simulink model "Supported_and_unsupported_combinations"  (Simulink 7.8)
settings: Solver=ode15s  StartTime=0.0  StopTime=inf  MaxStep=0.2  RelTol=1e-3
undefined symbols (not defined in the file): Engine, Engine1, Engine2, Engine3, Engine4, Engine5, Engine6, Engine7, Engine8, Engine9
libraries: sFunctionBlocks x32
(part 4 of 4)

== system Supported_and_unsupported_combinations/Engine8/IntakeManifold ==
  Mout : Inport
  inflow : Inport  Port=2
  IsothermalManifoldXO2 : S-Function  FunctionName=orsb_reservoir_isothermal_XO2  Parameters=V , R , Cp , pinit , XO2init ,  EnableBusSupport=off  mask(reservoir isothermal XO2 ){V=41.2801, R=288.4, Cp=1020, pinit=205590, XO2init=0.22}
      mask prompts: V "reservoir volume [l]"; R "gas constant [J/K/kg]"; Cp "fixed pressure spec heat [J/kg/K]"; pinit "initial pressure [Pa]"; XO2init "initial oxygen mass fraction [-]"
      mask help: Isothermal reservoir model with pressure and oxygen mass fraction as internal states.
      mask TabNameString: General ,General ,General ,Initialization ,Initialization
      mask Display:
      | port_label('input', 1, 'min ');
      | port_label('input', 2, 'mout ');
      | port_label('input', 3, 'Tin ');
      | port_label('input', 4, 'O2min ');
      | port_label('output', 1, 'pout ');
      | port_label('output', 2, 'XO2out ');
  Pim : Outport
  XO2out : Outport  Port=2
  outflow : Outport  Port=3
  tag scope: EngineIntakeManifold_OutletPressure=global
  wires:
  Mout/1 -> IsothermalManifoldXO2/2
  IsothermalManifoldXO2/1 -> Pim/1, [EngineIntakeManifold_OutletPressure]
  IsothermalManifoldXO2/2 -> XO2out/1
  inflow/1 -> outflow/1  "flow"
  [MixTotalInFlow_Massflow] -> IsothermalManifoldXO2/1
  [MixTotalInFlow_OxygenFlow] -> IsothermalManifoldXO2/4
  [MixTotalInFlow_MixtureTemperature] -> IsothermalManifoldXO2/3

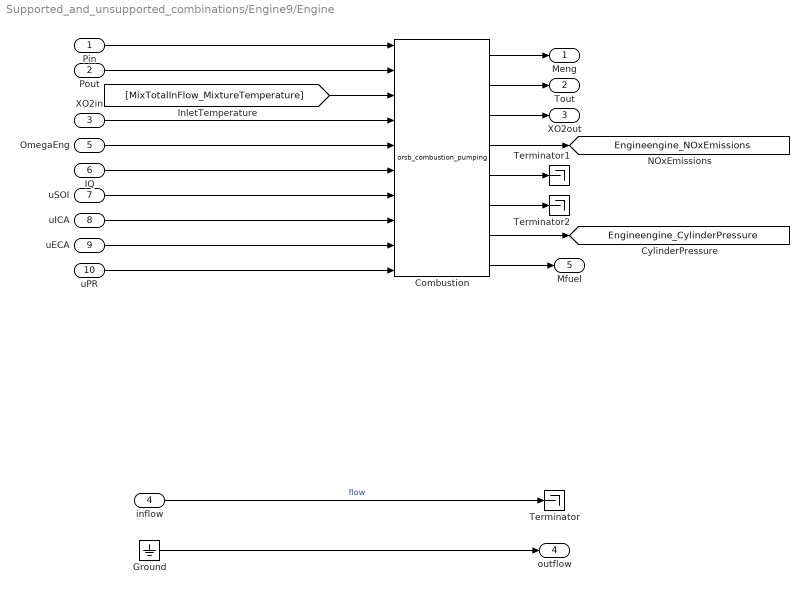
== system Supported_and_unsupported_combinations/Engine9/Engine ==
  Pin : Inport
  Pout : Inport  Port=2
  XO2in : Inport  Port=3
  inflow : Inport  Port=4
  OmegaEng : Inport  Port=5
  IQ : Inport  Port=6
  uSOI : Inport  Port=7
  uICA : Inport  Port=8
  uECA : Inport  Port=9
  uPR : Inport  Port=10
  Combustion : S-Function  FunctionName=orsb_combustion_pumping  Parameters=Displ, CompRatio, Ncyl, ValveMdl, TmpMdl, IgnitMdl, PressMdl, Cp, Cv, port_num_NOx, NOxMdl,  EnableBusSupport=off  mask(combustion_pumping){Displ=12.9, CompRatio=18, Ncyl=6, ValveMdl=[0.00961171539106083 -0.172384589641163], TmpMdl=[-0.025503095647334 0.175522235872159 0.0255043476751577 0.0373865335774022 0], IgnitMdl=[0.484351292851209 0.143524113288744 -0.055676015193126 -0.0109937044135945 -0.025686692856836], PressMdl=[5.48733176777509 -0.092135251339445 -0.0332005633970498 0.773921335537747], Cp=1500, Cv=1200, port_num_NOx=4, NOxMdl=[-0.0710772115732251 13.258266248882 2.53650929146028 -4.98871540780321 18.9690745540948 3.51983329140351 7.35640722696346 -29.5494146545499 -12.7663876549855 -0.0214097840965915 0.143608010417368 -1.21453634962735 0.541720620436424 -0.0774873942784366 -0.515304310267613]}
      mask prompts: Displ "displacement"; CompRatio "compression ratio"; Ncyl "number of cylinders"; ValveMdl "valve model"; TmpMdl "temperature model"; IgnitMdl "ignition model"; PressMdl "pressure model"; port_num_NOx "Model NOx output port number"; NOxMdl "NOx parameters"
      mask help: Combustion development
      mask TabNameString: geometry,geometry,geometry,thermodynamics,thermodynamics,thermodynamics,thermodynamics,thermodynamics,thermodynamics,NOx,NOx
      mask Display:
      | port_label('input', 1, 'Pi');
      | port_label('input', 2, 'Pe');
      | port_label('input', 3, 'Ti');
      | port_label('input', 4, 'O2i');
      | port_label('input', 5, 'Ne');
      | port_label('input', 6, 'iq');
      | port_label('input', 7, 'soi');
      | port_label('input', 8, 'ica');
      | port_label('input', 9, 'eca');
      | port_label('input', 10, 'Prail');
      | port_label('output', 1, 'M');
      | port_label('output', 2, 'Te');
      | port_label('output', 3, 'XO2e');
      | port_label('output', 4, 'NOx');
      | port_label('output', 5, 'lambda');
      | port_label('output', 6, 'phi_ign');
      | port_label('output', 7, 'Pcyl');
      | port_label('output', 8, 'Mf');
  Ground : Ground
  Terminator : Terminator
  Terminator1 : Terminator
  Terminator2 : Terminator
  Meng : Outport
  Tout : Outport  Port=2
  XO2out : Outport  Port=3
  outflow : Outport  Port=4
  Mfuel : Outport  Port=5
  tag scope: Engineengine_CylinderPressure=global, Engineengine_NOxEmissions=global
  wires:
  uSOI/1 -> Combustion/7
  [MixTotalInFlow_MixtureTemperature] -> Combustion/3
  Combustion/4 -> [Engineengine_NOxEmissions]
  XO2in/1 -> Combustion/4
  Combustion/3 -> XO2out/1
  Combustion/2 -> Tout/1
  Pout/1 -> Combustion/2
  Pin/1 -> Combustion/1
  OmegaEng/1 -> Combustion/5
  Ground/1 -> outflow/1
  inflow/1 -> Terminator/1  "flow"
  Combustion/1 -> Meng/1
  Combustion/5 -> Terminator1/1
  Combustion/6 -> Terminator2/1
  Combustion/7 -> [Engineengine_CylinderPressure]
  Combustion/8 -> Mfuel/1
  IQ/1 -> Combustion/6
  uICA/1 -> Combustion/8
  uECA/1 -> Combustion/9
  uPR/1 -> Combustion/10

== system Supported_and_unsupported_combinations/Engine9/ExhaustManifold ==
  Meng : Inport
  Tin : Inport  Port=2
  XO2in : Inport  Port=3
  inflow : Inport  Port=4
  Mfuel : Inport  Port=5
  Add4 : Sum
  AdiabaticManifoldXO2 : S-Function  FunctionName=orsb_reservoir_adiabatic_XO2  Parameters=V , R , Cp , pinit , Tinit , XO2init ,  EnableBusSupport=off  mask(reservoir adiabatic XO2 ){V=50, R=288.4, Cp=1135, pinit=247140, Tinit=720.22, XO2init=0.15}
      mask prompts: V "reservoir volume [l]"; R "gas constant [J/K/kg]"; Cp "fixed pressure spec heat [J/kg/K]"; pinit "initial pressure [Pa]"; Tinit "initial temperature [K]"; XO2init "initial oxygen mass fraction [-]"
      mask help: Adiabatic reservoir model with pressure, temperature, and oxygen mass fraction as internal states.
      mask TabNameString: General ,General ,General ,Initialization ,Initialization ,Initialization
      mask Display:
      | port_label('input', 1, 'min ');
      | port_label('input', 2, 'mout ');
      | port_label('input', 3, 'Tin ');
      | port_label('input', 4, 'O2min ');
      | port_label('output', 1, 'pout ');
      | port_label('output', 2, 'Tout ');
      | port_label('output', 3, 'XO2out ');
  Conversion_XO2_lambda : Fcn  Expr=u(1) / 0.231362 * (1 + 14.59) / (14.59 * (1 - u(1) / 0.231362))+1
  Product2 : Product  RndMeth=Zero
  Saturation : Saturate  UpperLimit=0.2313  LowerLimit=0
  Pout : Outport
  outflow : Outport  Port=2
  tag scope: EngineExhaustManifold_OutletLambda=global, EngineExhaustManifold_OutletOxygenFraction=global, EngineExhaustManifold_OutletPressure=global, EngineExhaustManifold_OutletTemperature=global
  wires:
  Conversion_XO2_lambda/1 -> [EngineExhaustManifold_OutletLambda]
  [FlowSplitterTotalOutFlow_Massflow] -> AdiabaticManifoldXO2/2
  Mfuel/1 -> Add4/1
  inflow/1 -> outflow/1  "flow"
  XO2in/1 -> Product2/2
  AdiabaticManifoldXO2/3 -> [EngineExhaustManifold_OutletOxygenFraction], Saturation/1
  Tin/1 -> AdiabaticManifoldXO2/3
  AdiabaticManifoldXO2/2 -> [EngineExhaustManifold_OutletTemperature]
  AdiabaticManifoldXO2/1 -> [EngineExhaustManifold_OutletPressure], Pout/1
  Meng/1 -> Add4/2
  Product2/1 -> AdiabaticManifoldXO2/4
  Add4/1 -> Product2/1, AdiabaticManifoldXO2/1
  Saturation/1 -> Conversion_XO2_lambda/1

== system Supported_and_unsupported_combinations/Engine9/IntakeManifold ==
  Mout : Inport
  inflow : Inport  Port=2
  IsothermalManifoldXO2 : S-Function  FunctionName=orsb_reservoir_isothermal_XO2  Parameters=V , R , Cp , pinit , XO2init ,  EnableBusSupport=off  mask(reservoir isothermal XO2 ){V=41.2801, R=288.4, Cp=1020, pinit=205590, XO2init=0.22}
      mask prompts: V "reservoir volume [l]"; R "gas constant [J/K/kg]"; Cp "fixed pressure spec heat [J/kg/K]"; pinit "initial pressure [Pa]"; XO2init "initial oxygen mass fraction [-]"
      mask help: Isothermal reservoir model with pressure and oxygen mass fraction as internal states.
      mask TabNameString: General ,General ,General ,Initialization ,Initialization
      mask Display:
      | port_label('input', 1, 'min ');
      | port_label('input', 2, 'mout ');
      | port_label('input', 3, 'Tin ');
      | port_label('input', 4, 'O2min ');
      | port_label('output', 1, 'pout ');
      | port_label('output', 2, 'XO2out ');
  Pim : Outport
  XO2out : Outport  Port=2
  outflow : Outport  Port=3
  tag scope: EngineIntakeManifold_OutletPressure=global
  wires:
  [MixTotalInFlow_MixtureTemperature] -> IsothermalManifoldXO2/3
  [MixTotalInFlow_OxygenFlow] -> IsothermalManifoldXO2/4
  [MixTotalInFlow_Massflow] -> IsothermalManifoldXO2/1
  inflow/1 -> outflow/1  "flow"
  IsothermalManifoldXO2/2 -> XO2out/1
  IsothermalManifoldXO2/1 -> [EngineIntakeManifold_OutletPressure], Pim/1
  Mout/1 -> IsothermalManifoldXO2/2

== system Supported_and_unsupported_combinations/FlowSplitter/OutFlow1 ==
  inflow : Inport
  Mout1 : Outport
  outflow : Outport  Port=2
  tag scope: none=global
  wires:
  inflow/1 -> outflow/1  "flow"
  [none] -> [none], Mout1/1

== system Supported_and_unsupported_combinations/FlowSplitter/OutFlow2 ==
  inflow : Inport
  Mout2 : Outport
  outflow : Outport  Port=2
  tag scope: none=global
  wires:
  [none] -> [none], Mout2/1
  inflow/1 -> outflow/1  "flow"

== system Supported_and_unsupported_combinations/FlowSplitter/TotalOutFlow ==
  Mout1 : Inport
  Mout2 : Inport  Port=2
  inflow : Inport  Port=3
  AuxiliaryManifold : sFunctionBlocks/AuxiliaryManifold  Tag=isAuxManifold  V=1  R=288  Cp=1020  pinit=1e5  isActive=0
  FlowSummation : Sum
  outflow : Outport
  tag scope: none=global
  wires:
  [none] -> AuxiliaryManifold/3
  [none] -> AuxiliaryManifold/1
  AuxiliaryManifold/1 -> [none]
  inflow/1 -> outflow/1  "flow"
  Mout1/1 -> FlowSummation/1
  Mout2/1 -> FlowSummation/2
  FlowSummation/1 -> AuxiliaryManifold/2, [none]

== system Supported_and_unsupported_combinations/FlowSplitter1/OutFlow1 ==
  inflow : Inport
  Mout1 : Outport
  outflow : Outport  Port=2
  tag scope: none=global
  wires:
  [none] -> Mout1/1, [none]
  inflow/1 -> outflow/1  "flow"

== system Supported_and_unsupported_combinations/FlowSplitter1/OutFlow2 ==
  inflow : Inport
  Mout2 : Outport
  outflow : Outport  Port=2
  tag scope: none=global
  wires:
  inflow/1 -> outflow/1  "flow"
  [none] -> Mout2/1, [none]

== system Supported_and_unsupported_combinations/FlowSplitter1/TotalOutFlow ==
  Mout1 : Inport
  Mout2 : Inport  Port=2
  inflow : Inport  Port=3
  AuxiliaryManifold : sFunctionBlocks/AuxiliaryManifold  Tag=isAuxManifold  V=1  R=288  Cp=1020  pinit=1e5  isActive=0
  FlowSummation : Sum
  outflow : Outport
  tag scope: none=global
  wires:
  FlowSummation/1 -> [none], AuxiliaryManifold/2
  Mout2/1 -> FlowSummation/2
  Mout1/1 -> FlowSummation/1
  inflow/1 -> outflow/1  "flow"
  AuxiliaryManifold/1 -> [none]
  [none] -> AuxiliaryManifold/1
  [none] -> AuxiliaryManifold/3

== system Supported_and_unsupported_combinations/FlowSplitter2/OutFlow1 ==
  inflow : Inport
  Mout1 : Outport
  outflow : Outport  Port=2
  tag scope: none=global
  wires:
  [none] -> Mout1/1, [none]
  inflow/1 -> outflow/1  "flow"

== system Supported_and_unsupported_combinations/FlowSplitter2/OutFlow2 ==
  inflow : Inport
  Mout2 : Outport
  outflow : Outport  Port=2
  tag scope: none=global
  wires:
  inflow/1 -> outflow/1  "flow"
  [none] -> Mout2/1, [none]

== system Supported_and_unsupported_combinations/FlowSplitter2/TotalOutFlow ==
  Mout1 : Inport
  Mout2 : Inport  Port=2
  inflow : Inport  Port=3
  AuxiliaryManifold : sFunctionBlocks/AuxiliaryManifold  Tag=isAuxManifold  V=1  R=288  Cp=1020  pinit=1e5  isActive=0
  FlowSummation : Sum
  outflow : Outport
  tag scope: none=global
  wires:
  FlowSummation/1 -> [none], AuxiliaryManifold/2
  Mout2/1 -> FlowSummation/2
  Mout1/1 -> FlowSummation/1
  inflow/1 -> outflow/1  "flow"
  AuxiliaryManifold/1 -> [none]
  [none] -> AuxiliaryManifold/1
  [none] -> AuxiliaryManifold/3

== system Supported_and_unsupported_combinations/FlowSplitter3/OutFlow1 ==
  inflow : Inport
  Mout1 : Outport
  outflow : Outport  Port=2
  tag scope: none=global
  wires:
  inflow/1 -> outflow/1  "flow"
  [none] -> [none], Mout1/1

== system Supported_and_unsupported_combinations/FlowSplitter3/OutFlow2 ==
  inflow : Inport
  Mout2 : Outport
  outflow : Outport  Port=2
  tag scope: none=global
  wires:
  [none] -> [none], Mout2/1
  inflow/1 -> outflow/1  "flow"

== system Supported_and_unsupported_combinations/FlowSplitter3/TotalOutFlow ==
  Mout1 : Inport
  Mout2 : Inport  Port=2
  inflow : Inport  Port=3
  AuxiliaryManifold : sFunctionBlocks/AuxiliaryManifold  Tag=isAuxManifold  V=1  R=288  Cp=1020  pinit=1e5  isActive=0
  FlowSummation : Sum
  outflow : Outport
  tag scope: none=global
  wires:
  [none] -> AuxiliaryManifold/3
  [none] -> AuxiliaryManifold/1
  AuxiliaryManifold/1 -> [none]
  inflow/1 -> outflow/1  "flow"
  Mout1/1 -> FlowSummation/1
  Mout2/1 -> FlowSummation/2
  FlowSummation/1 -> AuxiliaryManifold/2, [none]

== system Supported_and_unsupported_combinations/Mix/InFlow1 ==
  inflow : Inport
  Flow1 : Subsystem
  Tin : Outport
  Min : Outport  Port=2
  XO2in : Outport  Port=3
  outflow : Outport  Port=4
  wires:
  Flow1/3(XO2in) -> XO2in/1
  Flow1/2(Min) -> Min/1
  Flow1/1(Tin) -> Tin/1
  inflow/1 -> outflow/1  "flow"
  [none] -> Flow1/3(In3)
  [none] -> Flow1/2(In2)
  [none] -> Flow1/1(In1)

== system Supported_and_unsupported_combinations/Mix/InFlow2 ==
  inflow : Inport
  Flow2 : Subsystem
  Tin : Outport
  Min : Outport  Port=2
  XO2in : Outport  Port=3
  outflow : Outport  Port=4
  wires:
  Flow2/3(XO2in) -> XO2in/1
  Flow2/2(Min) -> Min/1
  Flow2/1(Tin) -> Tin/1
  inflow/1 -> outflow/1  "flow"
  [none] -> Flow2/3(In3)
  [none] -> Flow2/2(In2)
  [none] -> Flow2/1(In1)

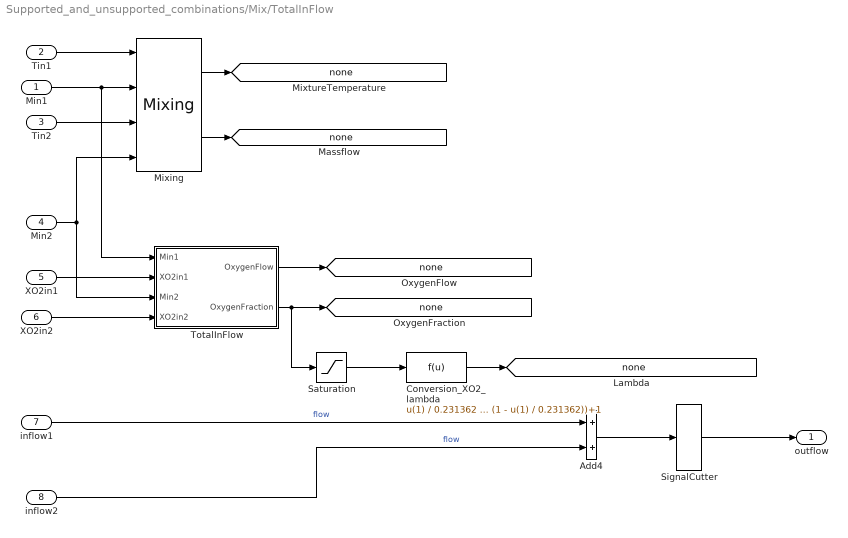
== system Supported_and_unsupported_combinations/Mix/TotalInFlow ==
  Min1 : Inport
  Tin1 : Inport  Port=2
  Tin2 : Inport  Port=3
  Min2 : Inport  Port=4
  XO2in1 : Inport  Port=5
  XO2in2 : Inport  Port=6
  inflow1 : Inport  Port=7
  inflow2 : Inport  Port=8
  Add4 : Sum
  Conversion_XO2_lambda : Fcn  Expr=u(1) / 0.231362 * (1 + 14.59) / (14.59 * (1 - u(1) / 0.231362))+1
  Mixing : sFunctionBlocks/Mixing  Cp1=1020.25  Cp2=1135.841
  Saturation : Saturate  UpperLimit=0.2313  LowerLimit=0
  SignalCutter : sFunctionBlocks/SignalCutter
  TotalInFlow : Subsystem
  outflow : Outport
  tag scope: none=global
  wires:
  SignalCutter/1 -> outflow/1
  Saturation/1 -> Conversion_XO2_lambda/1
  Conversion_XO2_lambda/1 -> [none]
  TotalInFlow/2(OxygenFraction) -> Saturation/1, [none]
  TotalInFlow/1(OxygenFlow) -> [none]
  inflow2/1 -> Add4/2  "flow"
  inflow1/1 -> Add4/1  "flow"
  Add4/1 -> SignalCutter/1
  XO2in2/1 -> TotalInFlow/4(XO2in2)
  XO2in1/1 -> TotalInFlow/2(XO2in1)
  Tin2/1 -> Mixing/3
  Tin1/1 -> Mixing/1
  Mixing/2 -> [none]
  Mixing/1 -> [none]
  Min2/1 -> TotalInFlow/3(Min2), Mixing/4
  Min1/1 -> TotalInFlow/1(Min1), Mixing/2

== system Supported_and_unsupported_combinations/Mix1/InFlow1 ==
  inflow : Inport
  Flow1 : Subsystem
  Tin : Outport
  Min : Outport  Port=2
  XO2in : Outport  Port=3
  outflow : Outport  Port=4
  wires:
  [none] -> Flow1/1(In1)
  [none] -> Flow1/2(In2)
  [none] -> Flow1/3(In3)
  inflow/1 -> outflow/1  "flow"
  Flow1/1(Tin) -> Tin/1
  Flow1/2(Min) -> Min/1
  Flow1/3(XO2in) -> XO2in/1

== system Supported_and_unsupported_combinations/Mix1/InFlow2 ==
  inflow : Inport
  Flow2 : Subsystem
  Tin : Outport
  Min : Outport  Port=2
  XO2in : Outport  Port=3
  outflow : Outport  Port=4
  wires:
  [none] -> Flow2/1(In1)
  [none] -> Flow2/2(In2)
  [none] -> Flow2/3(In3)
  inflow/1 -> outflow/1  "flow"
  Flow2/1(Tin) -> Tin/1
  Flow2/2(Min) -> Min/1
  Flow2/3(XO2in) -> XO2in/1

== system Supported_and_unsupported_combinations/Mix1/TotalInFlow ==
  Min1 : Inport
  Tin1 : Inport  Port=2
  Tin2 : Inport  Port=3
  Min2 : Inport  Port=4
  XO2in1 : Inport  Port=5
  XO2in2 : Inport  Port=6
  inflow1 : Inport  Port=7
  inflow2 : Inport  Port=8
  Add4 : Sum
  Conversion_XO2_lambda : Fcn  Expr=u(1) / 0.231362 * (1 + 14.59) / (14.59 * (1 - u(1) / 0.231362))+1
  Mixing : sFunctionBlocks/Mixing  Cp1=1020.25  Cp2=1135.841
  Saturation : Saturate  UpperLimit=0.2313  LowerLimit=0
  SignalCutter : sFunctionBlocks/SignalCutter
  TotalInFlow : Subsystem
  outflow : Outport
  tag scope: none=global
  wires:
  Min1/1 -> Mixing/2, TotalInFlow/1(Min1)
  Min2/1 -> Mixing/4, TotalInFlow/3(Min2)
  Mixing/1 -> [none]
  Mixing/2 -> [none]
  Tin1/1 -> Mixing/1
  Tin2/1 -> Mixing/3
  XO2in1/1 -> TotalInFlow/2(XO2in1)
  XO2in2/1 -> TotalInFlow/4(XO2in2)
  Add4/1 -> SignalCutter/1
  inflow1/1 -> Add4/1  "flow"
  inflow2/1 -> Add4/2  "flow"
  TotalInFlow/1(OxygenFlow) -> [none]
  TotalInFlow/2(OxygenFraction) -> [none], Saturation/1
  Conversion_XO2_lambda/1 -> [none]
  Saturation/1 -> Conversion_XO2_lambda/1
  SignalCutter/1 -> outflow/1

== system Supported_and_unsupported_combinations/Mix2/InFlow1 ==
  inflow : Inport
  Flow1 : Subsystem
  Tin : Outport
  Min : Outport  Port=2
  XO2in : Outport  Port=3
  outflow : Outport  Port=4
  wires:
  [none] -> Flow1/1(In1)
  [none] -> Flow1/2(In2)
  [none] -> Flow1/3(In3)
  inflow/1 -> outflow/1  "flow"
  Flow1/1(Tin) -> Tin/1
  Flow1/2(Min) -> Min/1
  Flow1/3(XO2in) -> XO2in/1

== system Supported_and_unsupported_combinations/Mix2/InFlow2 ==
  inflow : Inport
  Flow2 : Subsystem
  Tin : Outport
  Min : Outport  Port=2
  XO2in : Outport  Port=3
  outflow : Outport  Port=4
  wires:
  [none] -> Flow2/1(In1)
  [none] -> Flow2/2(In2)
  [none] -> Flow2/3(In3)
  inflow/1 -> outflow/1  "flow"
  Flow2/1(Tin) -> Tin/1
  Flow2/2(Min) -> Min/1
  Flow2/3(XO2in) -> XO2in/1

== system Supported_and_unsupported_combinations/Mix2/TotalInFlow ==
  Min1 : Inport
  Tin1 : Inport  Port=2
  Tin2 : Inport  Port=3
  Min2 : Inport  Port=4
  XO2in1 : Inport  Port=5
  XO2in2 : Inport  Port=6
  inflow1 : Inport  Port=7
  inflow2 : Inport  Port=8
  Add4 : Sum
  Conversion_XO2_lambda : Fcn  Expr=u(1) / 0.231362 * (1 + 14.59) / (14.59 * (1 - u(1) / 0.231362))+1
  Mixing : sFunctionBlocks/Mixing  Cp1=1020.25  Cp2=1135.841
  Saturation : Saturate  UpperLimit=0.2313  LowerLimit=0
  SignalCutter : sFunctionBlocks/SignalCutter
  TotalInFlow : Subsystem
  outflow : Outport
  tag scope: none=global
  wires:
  Min1/1 -> Mixing/2, TotalInFlow/1(Min1)
  Min2/1 -> Mixing/4, TotalInFlow/3(Min2)
  Mixing/1 -> [none]
  Mixing/2 -> [none]
  Tin1/1 -> Mixing/1
  Tin2/1 -> Mixing/3
  XO2in1/1 -> TotalInFlow/2(XO2in1)
  XO2in2/1 -> TotalInFlow/4(XO2in2)
  Add4/1 -> SignalCutter/1
  inflow1/1 -> Add4/1  "flow"
  inflow2/1 -> Add4/2  "flow"
  TotalInFlow/1(OxygenFlow) -> [none]
  TotalInFlow/2(OxygenFraction) -> [none], Saturation/1
  Conversion_XO2_lambda/1 -> [none]
  Saturation/1 -> Conversion_XO2_lambda/1
  SignalCutter/1 -> outflow/1

== system Supported_and_unsupported_combinations/Mix3/InFlow1 ==
  inflow : Inport
  Flow1 : Subsystem
  Tin : Outport
  Min : Outport  Port=2
  XO2in : Outport  Port=3
  outflow : Outport  Port=4
  wires:
  Flow1/3(XO2in) -> XO2in/1
  Flow1/2(Min) -> Min/1
  Flow1/1(Tin) -> Tin/1
  inflow/1 -> outflow/1  "flow"
  [none] -> Flow1/3(In3)
  [none] -> Flow1/2(In2)
  [none] -> Flow1/1(In1)

== system Supported_and_unsupported_combinations/Mix3/InFlow2 ==
  inflow : Inport
  Flow2 : Subsystem
  Tin : Outport
  Min : Outport  Port=2
  XO2in : Outport  Port=3
  outflow : Outport  Port=4
  wires:
  Flow2/3(XO2in) -> XO2in/1
  Flow2/2(Min) -> Min/1
  Flow2/1(Tin) -> Tin/1
  inflow/1 -> outflow/1  "flow"
  [none] -> Flow2/3(In3)
  [none] -> Flow2/2(In2)
  [none] -> Flow2/1(In1)

== system Supported_and_unsupported_combinations/Mix3/TotalInFlow ==
  Min1 : Inport
  Tin1 : Inport  Port=2
  Tin2 : Inport  Port=3
  Min2 : Inport  Port=4
  XO2in1 : Inport  Port=5
  XO2in2 : Inport  Port=6
  inflow1 : Inport  Port=7
  inflow2 : Inport  Port=8
  Add4 : Sum
  Conversion_XO2_lambda : Fcn  Expr=u(1) / 0.231362 * (1 + 14.59) / (14.59 * (1 - u(1) / 0.231362))+1
  Mixing : sFunctionBlocks/Mixing  Cp1=1020.25  Cp2=1135.841
  Saturation : Saturate  UpperLimit=0.2313  LowerLimit=0
  SignalCutter : sFunctionBlocks/SignalCutter
  TotalInFlow : Subsystem
  outflow : Outport
  tag scope: none=global
  wires:
  SignalCutter/1 -> outflow/1
  Saturation/1 -> Conversion_XO2_lambda/1
  Conversion_XO2_lambda/1 -> [none]
  TotalInFlow/2(OxygenFraction) -> Saturation/1, [none]
  TotalInFlow/1(OxygenFlow) -> [none]
  inflow2/1 -> Add4/2  "flow"
  inflow1/1 -> Add4/1  "flow"
  Add4/1 -> SignalCutter/1
  XO2in2/1 -> TotalInFlow/4(XO2in2)
  XO2in1/1 -> TotalInFlow/2(XO2in1)
  Tin2/1 -> Mixing/3
  Tin1/1 -> Mixing/1
  Mixing/2 -> [none]
  Mixing/1 -> [none]
  Min2/1 -> TotalInFlow/3(Min2), Mixing/4
  Min1/1 -> TotalInFlow/1(Min1), Mixing/2

== system Supported_and_unsupported_combinations/Mix/InFlow1/Flow1 ==
  In1 : Inport
  In2 : Inport  Port=2
  In3 : Inport  Port=3
  Tin : Outport
  Min : Outport  Port=2
  XO2in : Outport  Port=3
  wires:
  In3/1 -> XO2in/1
  In2/1 -> Min/1
  In1/1 -> Tin/1

== system Supported_and_unsupported_combinations/Mix/InFlow2/Flow2 ==
  In1 : Inport
  In2 : Inport  Port=2
  In3 : Inport  Port=3
  Tin : Outport
  Min : Outport  Port=2
  XO2in : Outport  Port=3
  wires:
  In3/1 -> XO2in/1
  In2/1 -> Min/1
  In1/1 -> Tin/1

== system Supported_and_unsupported_combinations/Mix/TotalInFlow/TotalInFlow ==
  Min1 : Inport
  XO2in1 : Inport  Port=2
  Min2 : Inport  Port=3
  XO2in2 : Inport  Port=4
  Add1 : Sum
  Add4 : Sum
  Divide : Product  Inputs=*/
  Product1 : Product  RndMeth=Zero
  Product2 : Product  RndMeth=Zero
  Saturation : Saturate  UpperLimit=inf  LowerLimit=0.000001
  OxygenFlow : Outport
  OxygenFraction : Outport  Port=2
  wires:
  Saturation/1 -> Divide/2
  Divide/1 -> OxygenFraction/1
  Add1/1 -> Saturation/1
  Product2/1 -> Add4/1
  Product1/1 -> Add4/2
  Min1/1 -> Add1/1, Product2/1
  Min2/1 -> Add1/2, Product1/1
  XO2in1/1 -> Product2/2
  Add4/1 -> Divide/1, OxygenFlow/1
  XO2in2/1 -> Product1/2

== system Supported_and_unsupported_combinations/Mix1/InFlow1/Flow1 ==
  In1 : Inport
  In2 : Inport  Port=2
  In3 : Inport  Port=3
  Tin : Outport
  Min : Outport  Port=2
  XO2in : Outport  Port=3
  wires:
  In1/1 -> Tin/1
  In2/1 -> Min/1
  In3/1 -> XO2in/1

== system Supported_and_unsupported_combinations/Mix1/InFlow2/Flow2 ==
  In1 : Inport
  In2 : Inport  Port=2
  In3 : Inport  Port=3
  Tin : Outport
  Min : Outport  Port=2
  XO2in : Outport  Port=3
  wires:
  In1/1 -> Tin/1
  In2/1 -> Min/1
  In3/1 -> XO2in/1

== system Supported_and_unsupported_combinations/Mix1/TotalInFlow/TotalInFlow ==
  Min1 : Inport
  XO2in1 : Inport  Port=2
  Min2 : Inport  Port=3
  XO2in2 : Inport  Port=4
  Add1 : Sum
  Add4 : Sum
  Divide : Product  Inputs=*/
  Product1 : Product  RndMeth=Zero
  Product2 : Product  RndMeth=Zero
  Saturation : Saturate  UpperLimit=inf  LowerLimit=0.000001
  OxygenFlow : Outport
  OxygenFraction : Outport  Port=2
  wires:
  XO2in2/1 -> Product1/2
  Add4/1 -> OxygenFlow/1, Divide/1
  XO2in1/1 -> Product2/2
  Min2/1 -> Product1/1, Add1/2
  Min1/1 -> Product2/1, Add1/1
  Product1/1 -> Add4/2
  Product2/1 -> Add4/1
  Add1/1 -> Saturation/1
  Divide/1 -> OxygenFraction/1
  Saturation/1 -> Divide/2

== system Supported_and_unsupported_combinations/Mix2/InFlow1/Flow1 ==
  In1 : Inport
  In2 : Inport  Port=2
  In3 : Inport  Port=3
  Tin : Outport
  Min : Outport  Port=2
  XO2in : Outport  Port=3
  wires:
  In1/1 -> Tin/1
  In2/1 -> Min/1
  In3/1 -> XO2in/1

== system Supported_and_unsupported_combinations/Mix2/InFlow2/Flow2 ==
  In1 : Inport
  In2 : Inport  Port=2
  In3 : Inport  Port=3
  Tin : Outport
  Min : Outport  Port=2
  XO2in : Outport  Port=3
  wires:
  In1/1 -> Tin/1
  In2/1 -> Min/1
  In3/1 -> XO2in/1

== system Supported_and_unsupported_combinations/Mix2/TotalInFlow/TotalInFlow ==
  Min1 : Inport
  XO2in1 : Inport  Port=2
  Min2 : Inport  Port=3
  XO2in2 : Inport  Port=4
  Add1 : Sum
  Add4 : Sum
  Divide : Product  Inputs=*/
  Product1 : Product  RndMeth=Zero
  Product2 : Product  RndMeth=Zero
  Saturation : Saturate  UpperLimit=inf  LowerLimit=0.000001
  OxygenFlow : Outport
  OxygenFraction : Outport  Port=2
  wires:
  XO2in2/1 -> Product1/2
  Add4/1 -> OxygenFlow/1, Divide/1
  XO2in1/1 -> Product2/2
  Min2/1 -> Product1/1, Add1/2
  Min1/1 -> Product2/1, Add1/1
  Product1/1 -> Add4/2
  Product2/1 -> Add4/1
  Add1/1 -> Saturation/1
  Divide/1 -> OxygenFraction/1
  Saturation/1 -> Divide/2

== system Supported_and_unsupported_combinations/Mix3/InFlow1/Flow1 ==
  In1 : Inport
  In2 : Inport  Port=2
  In3 : Inport  Port=3
  Tin : Outport
  Min : Outport  Port=2
  XO2in : Outport  Port=3
  wires:
  In3/1 -> XO2in/1
  In2/1 -> Min/1
  In1/1 -> Tin/1

== system Supported_and_unsupported_combinations/Mix3/InFlow2/Flow2 ==
  In1 : Inport
  In2 : Inport  Port=2
  In3 : Inport  Port=3
  Tin : Outport
  Min : Outport  Port=2
  XO2in : Outport  Port=3
  wires:
  In3/1 -> XO2in/1
  In2/1 -> Min/1
  In1/1 -> Tin/1

== system Supported_and_unsupported_combinations/Mix3/TotalInFlow/TotalInFlow ==
  Min1 : Inport
  XO2in1 : Inport  Port=2
  Min2 : Inport  Port=3
  XO2in2 : Inport  Port=4
  Add1 : Sum
  Add4 : Sum
  Divide : Product  Inputs=*/
  Product1 : Product  RndMeth=Zero
  Product2 : Product  RndMeth=Zero
  Saturation : Saturate  UpperLimit=inf  LowerLimit=0.000001
  OxygenFlow : Outport
  OxygenFraction : Outport  Port=2
  wires:
  Saturation/1 -> Divide/2
  Divide/1 -> OxygenFraction/1
  Add1/1 -> Saturation/1
  Product2/1 -> Add4/1
  Product1/1 -> Add4/2
  Min1/1 -> Add1/1, Product2/1
  Min2/1 -> Add1/2, Product1/1
  XO2in1/1 -> Product2/2
  Add4/1 -> Divide/1, OxygenFlow/1
  XO2in2/1 -> Product1/2
